simulink library "posAug_cl_old"  (R2022a)
settings: Solver=VariableStepAuto  StartTime=0.0  StopTime=10.0  RelTol=1e-3
undefined symbols (not defined in the file): aoaStart, elevSet, elevStart, env, FLIGHTCONTROLLER, fltCtrl, initializeBussesFromBlock, intSat, pathLaps, pathLapsYaw, posAug, rollAmp, rollFreq, rollPhase, sEstim, slfExitTime, thetaIGain, thetaPGain, vhcl, yawAmp, yawFreq, yawPhase
libraries: slpidlib x10, simulink x5, posAug_cl_new x4, velocityAngle_ul x4, dspsigops x3, pathFollowingCtrlAoATurb_cl x1, pathFollowingCtrlAoATurbCoef_cl x1, courseFollowLookAhead_cl x1, ctrlAllocMatrix3CompCoef_cl x1, eulAng2RotMat_ul x1, $bdroot x1, angleBtw2Vecs_ul x1
(part 1 of 3)
settings Model: Creator=jbfine  LastModifiedBy=jbfine

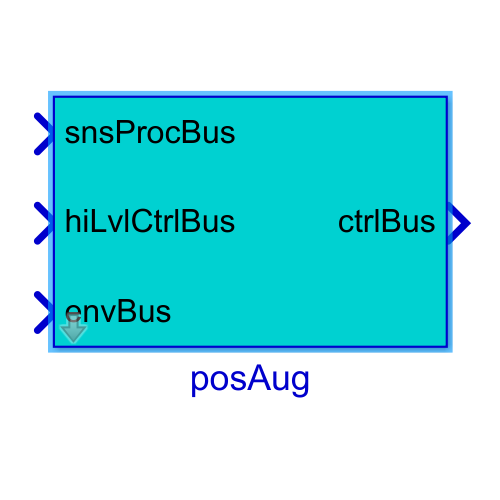
[thumbnail: Simulink's stored preview of the top-level diagram]
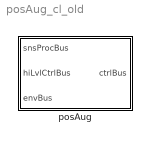
== system posAug_cl_old ==
  posAug : Subsystem  LoadFcn=initializeBussesFromBlock(gcb);  InitFcn=initializeBussesFromBlock(gcb);  VariantControl="strcmpi(FLIGHTCONTROLLER,\"posAug\")"  mask{initPosForInitSStar=vhcl.initPosVecGnd.Value, fluidDensity=env.water.density.Value, pathCtrl=fltCtrl, aeroStruct=vhcl.struct('OCT.aeroSurf')}
      mask prompts: initPosForInitSStar "Initial Position"; fluidDensity "Fluid Density"; pathCtrl "Controller"; aeroStruct "Aerodynamic Structure"
      settings: PreSaveFcn=initializeBussesFromBlock(gcb);
      mask DialogControl Container3 Prompt: courseFollow Params
      mask DialogControl Container4 Prompt: setpointToOutput Params

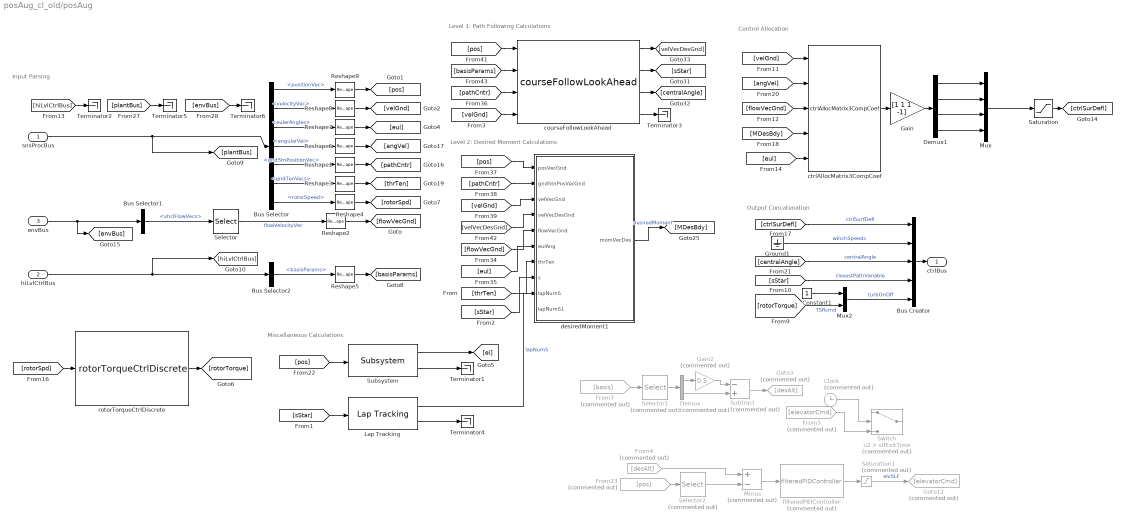
== system posAug_cl_old/posAug ==
  note: Level 2: Desired Moment Calculations
  note: Level 1: Path Following Calculations
  note: Input Parsing
  note: Miscellaneous Calculations
  note: Control Allocation
  note: Output Concatenation
  snsProcBus : Inport  OutDataTypeStr=Bus: sensorsProcessingBus
  hiLvlCtrlBus : Inport  Port=2  OutDataTypeStr=Bus: hiLvlCtrlBus
  envBus : Inport  Port=3  OutDataTypeStr=Bus: envBus
  Bus Creator : BusCreator  Inputs=5
  Bus Selector : BusSelector  OutputSignals=positionVec,velocityVec,eulerAngles,angularVel,gndStnPositionVec,gndTenVecs,rotorSpeed
  Bus Selector1 : BusSelector  OutputSignals=vhclFlowVecs
  Bus Selector2 : BusSelector  OutputSignals=basisParams
  Clock : Clock  Commented=on
  Constant1 : Constant
  Demux : Demux  Commented=on  Outputs=2
  Demux1 : Demux
  From23 : From  Commented=on  GotoTag=pos
  From4 : From  Commented=on  GotoTag=desAlt
  From5 : From  Commented=on  GotoTag=elevatorCmd
  From7 : From  Commented=on  GotoTag=basis
  Gain : Gain  Gain=[1 1 1 -1]
  Gain2 : Gain  Commented=on  Gain=0.5
  Goto12 : Goto  Commented=on  GotoTag=elevatorCmd
  Goto3 : Goto  Commented=on  GotoTag=desAlt
  Ground1 : Ground
  Lap Tracking : pathFollowingCtrlAoATurb_cl/pathFollowingCtrlAoATurb/Lap Tracking  SystemSampleTime=-1  VariantActivationTime=update diagram  Latency=0  AutoFrameSizeCalculation=off
  Minus : Sum  Commented=on  Inputs=+-
  Mux : Mux
  Mux2 : Mux  Inputs=2
  Reshape{1..9} (9 alike) : Reshape  OutputDimensionality=Column vector (2-D)
  Saturation : Saturate  UpperLimit=30  LowerLimit=-30
  Saturation1 : Saturate  Commented=on  UpperLimit=15  LowerLimit=-15
  Selector : Selector  NumberOfDimensions=2  InputPortWidth=3  IndexOptions=Select all,Index vector (dialog)  Indices=[1 3],5  OutputSizes=1,1
  Selector1 : Selector  Commented=on  InputPortWidth=5  IndexOptions=Index vector (dialog)  Indices=[2 3]  OutputSizes=1
  Selector2 : Selector  Commented=on  InputPortWidth=3  IndexOptions=Index vector (dialog)  Indices=3  OutputSizes=1
  Subsystem : pathFollowingCtrlAoATurbCoef_cl/pathFollowingCtrlAoATurbCoef/Subsystem  SystemSampleTime=-1  VariantActivationTime=update diagram  Latency=0  AutoFrameSizeCalculation=off
  Subtract : Sum  Commented=on  Inputs=-+
  Switch : Switch  Commented=on  Criteria=u2 > Threshold  Threshold=slfExitTime  SaturateOnIntegerOverflow=off  InputSameDT=off
  Terminator{1..6} (6 alike) : Terminator
  courseFollowLookAhead : courseFollowLookAhead_cl/courseFollowLookAhead  SystemSampleTime=-1  VariantActivationTime=update diagram  Latency=0  AutoFrameSizeCalculation=off
  ctrlAllocMatrix3CompCoef : ctrlAllocMatrix3CompCoef_cl/ctrlAllocMatrix3CompCoef  aeroStruct=vhcl.struct('OCT.aeroSurf')  fluidDensity=fluidDensity  arms=vhcl.struct('OCT.thrAttch')
  desiredMoment1 : Subsystem  AncestorBlock=pathFollowingCtrlAoATurb_cl/pathFollowingCtrlAoATurb/desiredMoment1
  filteredPIDController : filteredPIDController_ul/filteredPIDController  Commented=on  kp=elvKp  ki=elvKi  kd=elvKd  Value=1  externalReset=none
  rotorTorqueCtrlDiscrete : rotorTorqueCtrlDiscrete/rotorTorqueCtrlDiscrete  turb_struct=vhcl.struct('OCT.turb')  rho=rho
  ctrlBus : Outport  OutDataTypeStr=Bus: fltCtrlBus  VectorParamsAs1DForOutWhenUnconnected=off
  wires:
  [sStar] -> desiredMoment1/8(s)
  [eul] -> desiredMoment1/6(eulAng)
  [thrTen] -> desiredMoment1/7(thrTen)
  [pathCntr] -> desiredMoment1/2(gndStnPosVecGnd)
  [velGnd] -> desiredMoment1/3(velVecGnd)
  [pos] -> desiredMoment1/1(posVecGnd)
  desiredMoment1/1(momVecDes) -> [MDesBdy]  "desiredMoment"
  [velVecDesGnd] -> desiredMoment1/4(velVecDesGnd)
  [flowVecGnd] -> desiredMoment1/5(flowVecGnd)
  [velGnd] -> courseFollowLookAhead/4
  [pos] -> Subsystem/1
  Reshape7/1 -> [eul]
  [ctrlSurDefl] -> Bus Creator/1  "ctrlSurfDefl"
  courseFollowLookAhead/4 -> Terminator3/1
  [velGnd] -> ctrlAllocMatrix3CompCoef/1
  Gain/1 -> Demux1/1
  [eul] -> ctrlAllocMatrix3CompCoef/5
  [plantBus] -> Terminator5/1
  [envBus] -> Terminator6/1
  Saturation/1 -> [ctrlSurDefl]
  courseFollowLookAhead/1 -> [velVecDesGnd]
  [pos] -> courseFollowLookAhead/1
  Selector/1 -> Reshape2/1  "flowVelocityVec"
  ctrlAllocMatrix3CompCoef/1 -> Gain/1
  Reshape2/1 -> [flowVecGnd]
  Subsystem/1 -> [el]
  Bus Selector/7 -> Reshape4/1  "<rotorSpeed>"
  Constant1/1 -> Mux2/1
  Reshape1/1 -> [pathCntr]
  Bus Selector/6 -> Reshape3/1  "<gndTenVecs>"
  [angVel] -> ctrlAllocMatrix3CompCoef/2
  Reshape8/1 -> [velGnd]
  Subsystem/2 -> Terminator1/1
  Reshape3/1 -> [thrTen]
  [hiLvlCtrlBus] -> Terminator2/1
  Reshape6/1 -> [angVel]
  [flowVecGnd] -> ctrlAllocMatrix3CompCoef/3
  Reshape4/1 -> [rotorSpd]
  snsProcBus/1 -> Bus Selector/1, [plantBus]
  [rotorSpd] -> rotorTorqueCtrlDiscrete/1
  courseFollowLookAhead/3 -> [centralAngle]
  Mux2/1 -> Bus Creator/5  "turbOnOff"
  Reshape5/1 -> [basisParams]
  Bus Selector/4 -> Reshape6/1  "<angularVel>"
  Reshape9/1 -> [pos]
  Bus Selector/2 -> Reshape8/1  "<velocityVec>"
  Ground1/1 -> Bus Creator/2  "winchSpeeds"
  Bus Selector1/1 -> Selector/1  "<vhclFlowVecs>"
  Bus Selector/3 -> Reshape7/1  "<eulerAngles>"
  courseFollowLookAhead/2 -> [sStar]
  Bus Selector/1 -> Reshape9/1  "<positionVec>"
  hiLvlCtrlBus/1 -> Bus Selector2/1, [hiLvlCtrlBus]
  Bus Creator/1 -> ctrlBus/1
  [rotorTorque] -> Mux2/2  "TSRcmd"
  rotorTorqueCtrlDiscrete/1 -> [rotorTorque]
  Bus Selector2/1 -> Reshape5/1  "<basisParams>"
  envBus/1 -> Bus Selector1/1, [envBus]
  [basisParams] -> courseFollowLookAhead/2
  [sStar] -> Bus Creator/4  "closestPathVariable"
  [MDesBdy] -> ctrlAllocMatrix3CompCoef/4
  Bus Selector/5 -> Reshape1/1  "<gndStnPositionVec>"
  [centralAngle] -> Bus Creator/3  "centralAngle"
  [pathCntr] -> courseFollowLookAhead/3
  [sStar] -> Lap Tracking/1
  Lap Tracking/1 -> desiredMoment1/9(lapNumS)  "lapNumS"
  Lap Tracking/2 -> Terminator4/1
  Selector2/1 -> Minus/2
  Demux/1 -> Gain2/1
  Gain2/1 -> Subtract/1
  Demux/2 -> Subtract/2
  From4/1 -> Minus/1
  From23/1 -> Selector2/1
  Selector1/1 -> Demux/1
  From7/1 -> Selector1/1
  Subtract/1 -> Goto3/1
  From5/1 -> Switch/3
  Clock/1 -> Switch/2
  Demux1/1 -> Mux/1
  Demux1/4 -> Mux/4
  Demux1/2 -> Mux/2
  Mux/1 -> Saturation/1
  Minus/1 -> filteredPIDController/1
  filteredPIDController/1 -> Saturation1/1
  Saturation1/1 -> Goto12/1  "elvSLF"
  Demux1/3 -> Mux/3
